simulink library "csc_gib_gdn_inertial_burn_lib"  (R2015b)
settings: Solver=ode45  StartTime=0.0  StopTime=10.0  RelTol=1e-3
values from neighbouring files (symbols this model uses):
  csc_gdn_dt = fsw_dt    [csc_gdn_guidance_init.m]
  gdn_landing_targeting_max_alt = 1000.0    (= 1000)    [csc_gdn_guidance_init.m]
  gdn_millisec_per_cycle = csc_gdn_dt*1000    [csc_gib_gdn_inertial_burn_prep.m]
undefined symbols (not defined in the file or in its folder): accel, DiscIntNeverNeededParam, pos, q, vel
libraries: util_common_lib x17, simulink x12, util_frame_rotation_lib x4, simulink_extras x3, util_info_lib x2, csu_arg_aimpoint_roll_guidance_lib x2, util_fsw_frame_rotation_lib x2, util_quat_lib x1
settings Model: Creator=Nilesh  LastModifiedBy=Mark Agbayani
settings DataIOCC: SaveFormat=Array
settings DebuggingCC: UnderspecifiedInitializationDetection=Classic  MergeDetectMultiDrivingBlocksExec=none  SolverPrmCheckMsg=warning  StateNameClashWarn=warning
settings HardwareCC: ProdBitPerPointer=32  ProdLargestAtomicFloat=None  ProdIntDivRoundTo=Undefined  ProdEndianess=Unspecified  ProdWordSize=32  ProdHWDeviceType=32-bit Generic
settings GRTTargetCC: GeneratePreprocessorConditionals=Disable all
settings ConfigComp: CovModelRefEnable=Off  CovSFcnEnable=off

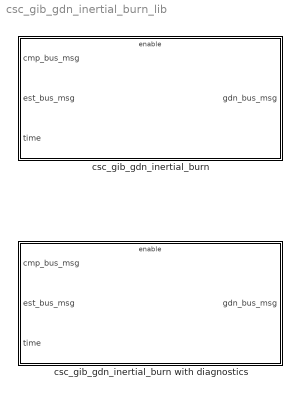
== system csc_gib_gdn_inertial_burn_lib ==
  csc_gib_gdn_inertial_burn : Subsystem
  csc_gib_gdn_inertial_burn with diagnostics : Subsystem

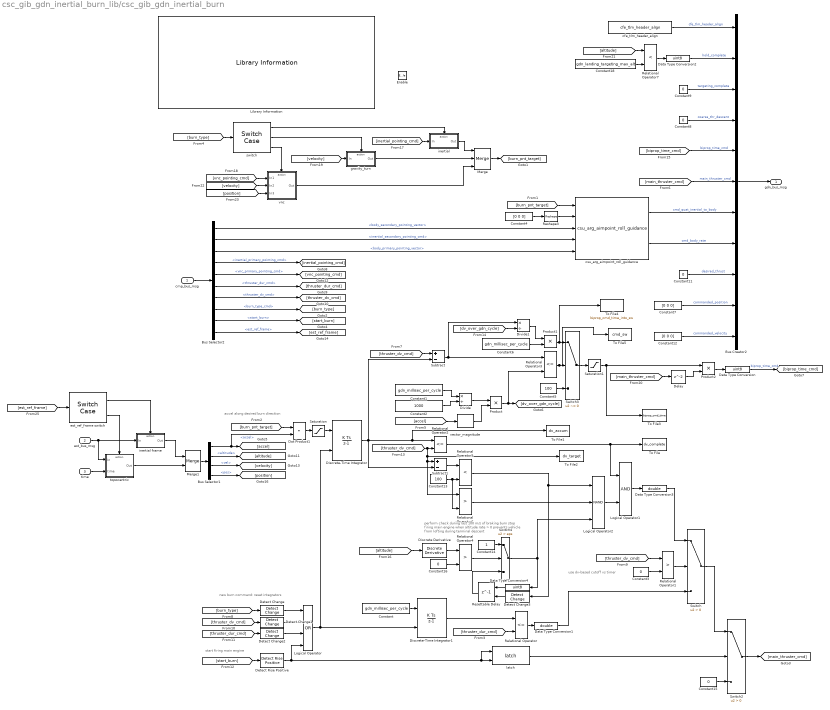
== system csc_gib_gdn_inertial_burn_lib/csc_gib_gdn_inertial_burn ==
  note: perform check during last 100 m/s of braking burn
      | stop firing main engine when altitude rate > 0
      | prevents vehicle from lofting during terminal descent
  note: use dv-based cutoff vs timer
  note: accel along desired burn direction
  note: new burn command: reset integrators
  note: start firing main engine
  cmp_bus_msg : Inport
  est_bus_msg : Inport  Port=2
  time : Inport  Port=3
  Enable : EnablePort  StatesWhenEnabling=reset
  Bus Selector1 : BusSelector  OutputSignals=accel,altitude,vel,pos
  Bus Selector2 : BusSelector  OutputSignals=body_secondary_pointing_vector,inertial_secondary_pointing_cmd,body_primary_pointing_vector,inertial_primary_pointing_cmd,vnc_primary_pointing_cmd,thruster_dur_cmd,thruster_dv_cmd,burn_type_cmd,start_burn,est_ref_frame
  Bus Creator2 : BusCreator  Inputs=11  OutDataTypeStr=Bus: gdn_bus_msg  NonVirtualBus=on
  Constant : Constant  Value=gdn_millisec_per_cycle
  Constant1 : Constant  Value=gdn_millisec_per_cycle
  Constant11 : Constant  Value=0
  Constant12 : Constant  Value=[0 0 0]
  Constant13 : Constant  Value=100
  Constant14 : Constant  OutDataTypeStr=uint8
  Constant15 : Constant  Value=0  OutDataTypeStr=double
  Constant16 : Constant  Value=0
  Constant18 : Constant  Value=gdn_landing_targeting_max_alt
  Constant2 : Constant  Value=1000
  Constant3 : Constant  Value=0
  Constant4 : Constant  Value=[0 0 0]
  Constant5 : Constant  Value=100
  Constant6 : Constant  Value=gdn_millisec_per_cycle
  Constant7 : Constant  Value=[0 0 0]
  Constant8 : Constant  Value=0  OutDataTypeStr=uint8
  Constant9 : Constant  Value=0  OutDataTypeStr=uint8
  Data Type Conversion : DataTypeConversion  OutDataTypeStr=uint8
  Data Type Conversion1 : DataTypeConversion  OutDataTypeStr=double
  Data Type Conversion2 : DataTypeConversion  OutDataTypeStr=uint8
  Data Type Conversion3 : DataTypeConversion  OutDataTypeStr=double
  Data Type Conversion4 : DataTypeConversion  OutDataTypeStr=uint8
  Delay : Delay
  Detect Change : simulink/Logic and Bit Operations/Detect Change  vinit=0  InputProcessing=Inherited  OutDataTypeStr=boolean
  Detect Change1 : simulink/Logic and Bit Operations/Detect Change  vinit=0  InputProcessing=Inherited  OutDataTypeStr=boolean
  Detect Change2 : simulink/Logic and Bit Operations/Detect Change  vinit=0  InputProcessing=Inherited  OutDataTypeStr=boolean
  Detect Change3 : simulink/Logic and Bit Operations/Detect Change  vinit=0  InputProcessing=Inherited  OutDataTypeStr=uint8
  Detect Rise Positive : simulink/Logic and Bit Operations/Detect Rise Positive  vinit=0  InputProcessing=Inherited  OutDataTypeStr=boolean
  Discrete Derivative : simulink/Discrete/Discrete Derivative  gainval=1.0  ICPrevScaledInput=0.0  InputProcessing=Inherited  OutMin=[]  OutMax=[]  OutDataType=fixdt(1, 16)  OutScaling=2^-10  DoSatur=off
  Discrete-Time Integrator : DiscreteIntegrator  ExternalReset=rising  SampleTime=csc_gdn_dt  ICPrevOutput=DiscIntNeverNeededParam  ICPrevScaledInput=DiscIntNeverNeededParam
  Discrete-Time Integrator1 : DiscreteIntegrator  ExternalReset=rising  SampleTime=csc_gdn_dt  ICPrevOutput=DiscIntNeverNeededParam  ICPrevScaledInput=DiscIntNeverNeededParam
  Divide : Product  Inputs=*/
  Divide1 : Product  Inputs=*/
  Dot Product1 : DotProduct  InputSameDT=on  OutDataTypeStr=Inherit: Inherit via internal rule
  Library Information : util_info_lib/Library Information  owner='jkaidy'
  Logical Operator : Logic  Operator=OR  Inputs=4  AllPortsSameDT=off  OutDataTypeStr=boolean
  Logical Operator1 : Logic  AllPortsSameDT=off  OutDataTypeStr=boolean
  Logical Operator2 : Logic  Operator=NAND  Inputs=3  AllPortsSameDT=off  OutDataTypeStr=boolean
  Merge : Merge  Inputs=3  InitialOutput=[0 0 1]
  Merge1 : Merge  InitialOutput=0
  Product : Product
  Product1 : Product
  Product2 : Product
  Relational Operator : RelationalOperator  Operator=<=  OutDataTypeStr=boolean
  Relational Operator1 : RelationalOperator  Operator=>  OutDataTypeStr=boolean
  Relational Operator2 : RelationalOperator  Operator=<=  OutDataTypeStr=boolean
  Relational Operator3 : RelationalOperator  Operator=<=  OutDataTypeStr=boolean
  Relational Operator4 : RelationalOperator  Operator=>  OutDataTypeStr=boolean
  Relational Operator5 : RelationalOperator  Operator=<  OutDataTypeStr=boolean
  Relational Operator6 : RelationalOperator  Operator=>  OutDataTypeStr=boolean
  Relational Operator7 : RelationalOperator  Operator=<  OutDataTypeStr=boolean
  Resettable Delay : Delay  DelayLength=1  InitialCondition=0  ExternalReset=Rising
      settings: InputPortMap=u0,r5
  Reshape3 : Reshape  OutputDimensionality=Column vector (2-D)
  Saturation : Saturate  UpperLimit=1e6  LowerLimit=0
  Saturation1 : Saturate  UpperLimit=100  LowerLimit=0
  Subtract : Sum  Inputs=+-
  Subtract1 : Sum  Inputs=+-
  Switch : Switch  Criteria=u2 > Threshold
  Switch2 : Switch  Criteria=u2 > Threshold
  Switch3 : Switch  Criteria=u2 ~= 0
  Switch4 : Switch  Criteria=u2 > Threshold  Threshold=eps
  To File : ToFile  Filename=dv_complete  MatrixName=dv_complete  SaveFormat=Timeseries
  To File1 : ToFile  Filename=dv_accum  MatrixName=dv_accum  SaveFormat=Timeseries
  To File2 : ToFile  Filename=dv_target  MatrixName=dv_target  SaveFormat=Timeseries
  To File3 : ToFile  Filename=biprop_cmd_time  MatrixName=biprop_cmd_time  SaveFormat=Timeseries
  To File4 : ToFile  Filename=biprop_cmd_time_into_sw  MatrixName=biprop_cmd_time_into_sw  SaveFormat=Timeseries
  To File5 : ToFile  Filename=cmd_sw  MatrixName=cmd_sw  SaveFormat=Timeseries
  cfe_tlm_header_align : util_common_lib/cfe_tlm_header_align
  csu_arg_aimpoint_roll_guidance : csu_arg_aimpoint_roll_guidance_lib/csu_arg_aimpoint_roll_guidance
  est_ref_frame switch : SwitchCase  CaseConditions={uint8(enum_reference_frame.inertial),uint8(enum_reference_frame.topocentric)}  ShowDefaultCase=off
  gravity_turn : Subsystem  TreatAsAtomicUnit=on
  inertial : Subsystem  TreatAsAtomicUnit=on
  inertial frame : Subsystem  TreatAsAtomicUnit=on
  latch : util_common_lib/latch  Initial_Latch=0
  switch : SwitchCase  CaseConditions={uint8(enum_burn_type.inertial),uint8(enum_burn_type.gravity_turn),uint8(enum_burn_type.vnc)}  ShowDefaultCase=off
  topocentric : Subsystem  TreatAsAtomicUnit=on
  vector_magnitude : util_common_lib/vector_magnitude  SystemSampleTime=-1
  vnc : Subsystem  TreatAsAtomicUnit=on
  gdn_bus_msg : Outport  OutDataTypeStr=Bus: gdn_bus_msg
  wires:
  Merge/1 -> [burn_pnt_target]
  Bus Selector2/4 -> [inertial_pointing_cmd]  "<inertial_primary_pointing_cmd>"
  Bus Selector2/5 -> [vnc_pointing_cmd]  "<vnc_primary_pointing_cmd>"
  [vnc_pointing_cmd] -> vnc/1(In1)
  [inertial_pointing_cmd] -> inertial/1(In)
  [burn_type] -> switch/1
  switch/3 -> vnc/Action
  inertial/1(Out) -> Merge/1
  switch/2 -> gravity_turn/Action
  gravity_turn/1(Out) -> Merge/2
  [velocity] -> gravity_turn/1(In)
  switch/1 -> inertial/Action
  Relational Operator7/1 -> Data Type Conversion2/1
  [altitude] -> Relational Operator7/1
  Constant18/1 -> Relational Operator7/2
  Bus Selector1/3 -> [velocity]  "<vel>"
  Data Type Conversion4/1 -> Resettable Delay/1
  Switch4/1 -> Data Type Conversion4/1, Logical Operator2/3
  latch/1 -> Switch2/2
  Resettable Delay/1 -> Switch4/3
  Detect Change3/1 -> Resettable Delay/2
  Constant14/1 -> Switch4/1
  Data Type Conversion3/1 -> Switch/1
  Relational Operator4/1 -> Switch4/2
  Bus Selector1/2 -> [altitude]  "<altitude>"
  Relational Operator6/1 -> Logical Operator2/2
  Discrete Derivative/1 -> Relational Operator4/1
  [altitude] -> Discrete Derivative/1
  Constant16/1 -> Relational Operator4/2
  Relational Operator5/1 -> Detect Change3/1, Logical Operator2/1
  Subtract1/1 -> Relational Operator5/1
  Constant13/1 -> Relational Operator5/2, Relational Operator6/2
  Discrete-Time Integrator/1 -> Subtract/2, To File1/1, Relational Operator2/1, Subtract1/2
  Logical Operator1/1 -> Data Type Conversion3/1
  Logical Operator2/1 -> Logical Operator1/2
  Switch2/1 -> [main_thruster_cmd]
  Constant15/1 -> Switch2/3
  Switch/1 -> Switch2/1
  Logical Operator/1 -> Discrete-Time Integrator1/2, Discrete-Time Integrator/2
  Detect Change2/1 -> Logical Operator/3
  Detect Change1/1 -> Logical Operator/2
  Detect Change/1 -> Logical Operator/1
  [thruster_dur_cmd] -> Detect Change2/1
  [thruster_dv_cmd] -> Detect Change1/1
  [burn_type] -> Detect Change/1
  [thruster_dv_cmd] -> Relational Operator1/1
  Relational Operator/1 -> Data Type Conversion1/1
  Constant3/1 -> Relational Operator1/2
  Data Type Conversion1/1 -> Switch/3
  Merge1/1 -> Bus Selector1/1
  [thruster_dv_cmd] -> Subtract1/1, Relational Operator6/1, To File2/1, Relational Operator2/2
  Relational Operator2/1 -> To File/1, Logical Operator1/1
  [thruster_dur_cmd] -> Relational Operator/2
  Dot Product1/1 -> Saturation/1
  Bus Selector1/1 -> [accel], Dot Product1/2  "<accel>"
  Discrete-Time Integrator1/1 -> Relational Operator/1
  Constant/1 -> Discrete-Time Integrator1/1
  [burn_pnt_target] -> Dot Product1/1
  Relational Operator1/1 -> Switch/2
  [start_burn] -> Detect Rise Positive/1
  Detect Rise Positive/1 -> Logical Operator/4, latch/2, latch/1
  Saturation/1 -> Discrete-Time Integrator/1
  [thruster_dv_cmd] -> Subtract/1
  Constant1/1 -> Divide/1
  Constant2/1 -> Divide/2
  Divide/1 -> Product/1
  [accel] -> vector_magnitude/1
  Product/1 -> Relational Operator3/2, [dv_over_gdn_cycle]
  Subtract/1 -> Divide1/1, Relational Operator3/1
  Relational Operator3/1 -> To File5/1, Switch3/2
  Constant5/1 -> Switch3/3
  [dv_over_gdn_cycle] -> Divide1/2
  Constant6/1 -> Product1/2
  Divide1/1 -> Product1/1
  Product1/1 -> To File4/1, Switch3/1
  Switch3/1 -> Saturation1/1
  vector_magnitude/1 -> Product/2
  Saturation1/1 -> Product2/1, To File3/1
  Data Type Conversion/1 -> [biprop_time_cmd]  "biprop_time_cmd"
  Constant7/1 -> Bus Creator2/10  "commanded_position"
  Constant12/1 -> Bus Creator2/11  "commanded_velocity"
  cfe_tlm_header_align/1 -> Bus Creator2/1  "cfe_tlm_header_align"
  Constant9/1 -> Bus Creator2/3  "targeting_complete"
  Data Type Conversion2/1 -> Bus Creator2/2  "hold_complete"
  csu_arg_aimpoint_roll_guidance/2 -> Bus Creator2/8  "cmd_body_rate"
  csu_arg_aimpoint_roll_guidance/1 -> Bus Creator2/7  "cmd_quat_inertial_to_body"
  Bus Creator2/1 -> gdn_bus_msg/1
  [main_thruster_cmd] -> Bus Creator2/6  "main_thruster_cmd"
  Constant8/1 -> Bus Creator2/4  "coarse_thr_descent"
  Constant11/1 -> Bus Creator2/9  "desired_thrust"
  Bus Selector2/9 -> [start_burn]  "<start_burn>"
  Bus Selector2/8 -> [burn_type]  "<burn_type_cmd>"
  Constant4/1 -> Reshape3/1
  Reshape3/1 -> csu_arg_aimpoint_roll_guidance/2
  Bus Selector2/3 -> csu_arg_aimpoint_roll_guidance/5  "<body_primary_pointing_vector>"
  Bus Selector2/2 -> csu_arg_aimpoint_roll_guidance/4  "<inertial_secondary_pointing_cmd>"
  Bus Selector2/1 -> csu_arg_aimpoint_roll_guidance/3  "<body_secondary_pointing_vector>"
  Bus Selector2/6 -> [thruster_dur_cmd]  "<thruster_dur_cmd>"
  Bus Selector2/7 -> [thruster_dv_cmd]  "<thruster_dv_cmd>"
  cmp_bus_msg/1 -> Bus Selector2/1
  [burn_pnt_target] -> csu_arg_aimpoint_roll_guidance/1
  [biprop_time_cmd] -> Bus Creator2/5  "biprop_time_cmd"
  vnc/1(Out) -> Merge/3
  time/1 -> topocentric/2(time)
  est_ref_frame switch/2 -> topocentric/Action
  topocentric/1(Out) -> Merge1/2
  inertial frame/1(Out) -> Merge1/1
  est_bus_msg/1 -> topocentric/1(In), inertial frame/1(In)
  est_ref_frame switch/1 -> inertial frame/Action
  [est_ref_frame] -> est_ref_frame switch/1
  Bus Selector2/10 -> [est_ref_frame]  "<est_ref_frame>"
  [position] -> vnc/3(In3)
  [velocity] -> vnc/2(In2)
  Bus Selector1/4 -> [position]  "<pos>"
  [main_thruster_cmd] -> Delay/1
  Delay/1 -> Product2/2
  Product2/1 -> Data Type Conversion/1

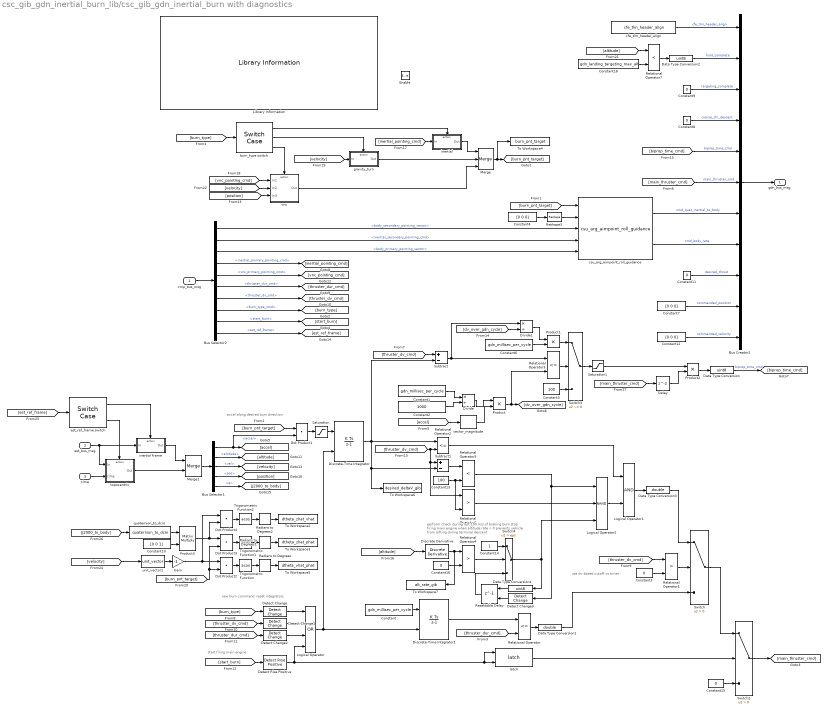
== system csc_gib_gdn_inertial_burn_lib/csc_gib_gdn_inertial_burn with diagnostics ==
  note: start firing main engine
  note: new burn command: reset integrators
  note: accel along desired burn direction
  note: use dv-based cutoff vs timer
  note: perform check during last 100 m/s of braking burn
      | stop firing main engine when altitude rate > 0
      | prevents vehicle from lofting during terminal descent
  cmp_bus_msg : Inport
  est_bus_msg : Inport  Port=2
  time : Inport  Port=3
  Enable : EnablePort  StatesWhenEnabling=reset
  Bus Selector1 : BusSelector  OutputSignals=accel,altitude,vel,pos,q
  Bus Selector2 : BusSelector  OutputSignals=body_secondary_pointing_vector,inertial_secondary_pointing_cmd,body_primary_pointing_vector,inertial_primary_pointing_cmd,vnc_primary_pointing_cmd,thruster_dur_cmd,thruster_dv_cmd,burn_type_cmd,start_burn,est_ref_frame
  Bus Creator2 : BusCreator  Inputs=11  OutDataTypeStr=Bus: gdn_bus_msg  NonVirtualBus=on
  Constant : Constant  Value=gdn_millisec_per_cycle
  Constant1 : Constant  Value=gdn_millisec_per_cycle
  Constant10 : Constant  Value=[0 0 1]
  Constant11 : Constant  Value=0
  Constant12 : Constant  Value=[0 0 0]
  Constant13 : Constant  Value=100
  Constant14 : Constant  OutDataTypeStr=uint8
  Constant15 : Constant  Value=0  OutDataTypeStr=double
  Constant16 : Constant  Value=0
  Constant18 : Constant  Value=gdn_landing_targeting_max_alt
  Constant2 : Constant  Value=1000
  Constant3 : Constant  Value=0
  Constant4 : Constant  Value=[0 0 0]
  Constant5 : Constant  Value=100
  Constant6 : Constant  Value=gdn_millisec_per_cycle
  Constant7 : Constant  Value=[0 0 0]
  Constant8 : Constant  Value=0  OutDataTypeStr=uint8
  Constant9 : Constant  Value=0  OutDataTypeStr=uint8
  Data Type Conversion : DataTypeConversion  OutDataTypeStr=uint8
  Data Type Conversion1 : DataTypeConversion  OutDataTypeStr=double
  Data Type Conversion2 : DataTypeConversion  OutDataTypeStr=uint8
  Data Type Conversion3 : DataTypeConversion  OutDataTypeStr=double
  Data Type Conversion4 : DataTypeConversion  OutDataTypeStr=uint8
  Delay : Delay
  Detect Change : simulink/Logic and Bit Operations/Detect Change  vinit=0  InputProcessing=Inherited  OutDataTypeStr=boolean
  Detect Change1 : simulink/Logic and Bit Operations/Detect Change  vinit=0  InputProcessing=Inherited  OutDataTypeStr=boolean
  Detect Change2 : simulink/Logic and Bit Operations/Detect Change  vinit=0  InputProcessing=Inherited  OutDataTypeStr=boolean
  Detect Change3 : simulink/Logic and Bit Operations/Detect Change  vinit=0  InputProcessing=Inherited  OutDataTypeStr=uint8
  Detect Rise Positive : simulink/Logic and Bit Operations/Detect Rise Positive  vinit=0  InputProcessing=Inherited  OutDataTypeStr=boolean
  Discrete Derivative : simulink/Discrete/Discrete Derivative  gainval=1.0  ICPrevScaledInput=0.0  InputProcessing=Inherited  OutMin=[]  OutMax=[]  OutDataType=fixdt(1, 16)  OutScaling=2^-10  DoSatur=off
  Discrete-Time Integrator : DiscreteIntegrator  ExternalReset=rising  SampleTime=csc_gdn_dt  ICPrevOutput=DiscIntNeverNeededParam  ICPrevScaledInput=DiscIntNeverNeededParam
  Discrete-Time Integrator1 : DiscreteIntegrator  ExternalReset=rising  SampleTime=csc_gdn_dt  ICPrevOutput=DiscIntNeverNeededParam  ICPrevScaledInput=DiscIntNeverNeededParam
  Divide : Product  Inputs=*/
  Divide1 : Product  Inputs=*/
  Dot Product{1..4} (4 alike) : DotProduct  InputSameDT=on  OutDataTypeStr=Inherit: Inherit via internal rule
  Gain : Gain  Gain=-1
  Library Information : util_info_lib/Library Information  owner='jkaidy'
  Logical Operator : Logic  Operator=OR  Inputs=4  AllPortsSameDT=off  OutDataTypeStr=boolean
  Logical Operator1 : Logic  AllPortsSameDT=off  OutDataTypeStr=boolean
  Logical Operator2 : Logic  Operator=NAND  Inputs=3  AllPortsSameDT=off  OutDataTypeStr=boolean
  Merge : Merge  Inputs=3  InitialOutput=[0 0 1]
  Merge1 : Merge  InitialOutput=0
  Product : Product
  Product1 : Product
  Product2 : Product
  Product3 : Product  Multiplication=Matrix(*)  RndMeth=Zero
  Radians to Degrees : simulink_extras/Transformations/Radians to Degrees
  Radians to Degrees1 : simulink_extras/Transformations/Radians to Degrees
  Radians to Degrees2 : simulink_extras/Transformations/Radians to Degrees
  Relational Operator : RelationalOperator  Operator=<=  OutDataTypeStr=boolean
  Relational Operator1 : RelationalOperator  Operator=>  OutDataTypeStr=boolean
  Relational Operator2 : RelationalOperator  Operator=<=  OutDataTypeStr=boolean
  Relational Operator3 : RelationalOperator  Operator=<=  OutDataTypeStr=boolean
  Relational Operator4 : RelationalOperator  Operator=>  OutDataTypeStr=boolean
  Relational Operator5 : RelationalOperator  Operator=<  OutDataTypeStr=boolean
  Relational Operator6 : RelationalOperator  Operator=>  OutDataTypeStr=boolean
  Relational Operator7 : RelationalOperator  Operator=<  OutDataTypeStr=boolean
  Resettable Delay : Delay  DelayLength=1  InitialCondition=0  ExternalReset=Rising
      settings: InputPortMap=u0,r5
  Reshape3 : Reshape  OutputDimensionality=Column vector (2-D)
  Saturation : Saturate  UpperLimit=1e6  LowerLimit=0
  Saturation1 : Saturate  UpperLimit=100  LowerLimit=0
  Subtract : Sum  Inputs=+-
  Subtract1 : Sum  Inputs=+-
  Switch : Switch  Criteria=u2 > Threshold
  Switch2 : Switch  Criteria=u2 > Threshold
  Switch3 : Switch  Criteria=u2 ~= 0
  Switch4 : Switch  Criteria=u2 > Threshold  Threshold=eps
  To Workspace2 : ToWorkspace  VariableName=dtheta_zhat_vhat  SaveFormat=Structure With Time  SampleTime=-1
  To Workspace3 : ToWorkspace  VariableName=dtheta_zhat_phat  SaveFormat=Structure With Time  SampleTime=-1
  To Workspace4 : ToWorkspace  VariableName=burn_pnt_target  SaveFormat=Structure With Time  SampleTime=-1
  To Workspace5 : ToWorkspace  VariableName=dtheta_vhat_phat  SaveFormat=Structure With Time  SampleTime=-1
  To Workspace6 : ToWorkspace  VariableName=desired_deltaV_gib  SaveFormat=Structure With Time  SampleTime=-1
  To Workspace7 : ToWorkspace  VariableName=alt_rate_gib  SaveFormat=Structure With Time  SampleTime=-1
  Trigonometric Function : Trigonometry  Operator=acos
  Trigonometric Function1 : Trigonometry  Operator=acos
  Trigonometric Function2 : Trigonometry  Operator=acos
  burn_type switch : SwitchCase  CaseConditions={uint8(enum_burn_type.inertial),uint8(enum_burn_type.gravity_turn),uint8(enum_burn_type.vnc)}  ShowDefaultCase=off
  cfe_tlm_header_align : util_common_lib/cfe_tlm_header_align
  csu_arg_aimpoint_roll_guidance : csu_arg_aimpoint_roll_guidance_lib/csu_arg_aimpoint_roll_guidance
  est_ref_frame switch : SwitchCase  CaseConditions={uint8(enum_reference_frame.inertial),uint8(enum_reference_frame.topocentric)}  ShowDefaultCase=off
  gravity_turn : Subsystem  TreatAsAtomicUnit=on
  inertial : Subsystem  TreatAsAtomicUnit=on
  inertial frame : Subsystem  TreatAsAtomicUnit=on
  latch : util_common_lib/latch  Initial_Latch=0
  quaternion_to_dcm : util_quat_lib/quaternion_to_dcm  SystemSampleTime=-1
  topocentric : Subsystem  TreatAsAtomicUnit=on
  unit_vector1 : util_common_lib/unit_vector  SystemSampleTime=-1
  vector_magnitude : util_common_lib/vector_magnitude  SystemSampleTime=-1
  vnc : Subsystem  TreatAsAtomicUnit=on
  gdn_bus_msg : Outport  OutDataTypeStr=Bus: gdn_bus_msg
  wires:
  Product2/1 -> Data Type Conversion/1
  Delay/1 -> Product2/2
  [main_thruster_cmd] -> Delay/1
  Data Type Conversion/1 -> [biprop_time_cmd]  "biprop_time_cmd"
  Saturation1/1 -> Product2/1
  Bus Selector1/5 -> [J2000_to_body]  "<q>"
  [velocity] -> vnc/2(In2)
  [position] -> vnc/3(In3)
  Bus Selector1/4 -> [position]  "<pos>"
  vnc/1(Out) -> Merge/3
  [biprop_time_cmd] -> Bus Creator2/5  "biprop_time_cmd"
  [burn_pnt_target] -> csu_arg_aimpoint_roll_guidance/1
  cmp_bus_msg/1 -> Bus Selector2/1
  Bus Selector2/7 -> [thruster_dv_cmd]  "<thruster_dv_cmd>"
  Bus Selector2/6 -> [thruster_dur_cmd]  "<thruster_dur_cmd>"
  Bus Selector2/1 -> csu_arg_aimpoint_roll_guidance/3  "<body_secondary_pointing_vector>"
  Bus Selector2/2 -> csu_arg_aimpoint_roll_guidance/4  "<inertial_secondary_pointing_cmd>"
  Bus Selector2/3 -> csu_arg_aimpoint_roll_guidance/5  "<body_primary_pointing_vector>"
  Reshape3/1 -> csu_arg_aimpoint_roll_guidance/2
  Constant4/1 -> Reshape3/1
  Bus Selector2/8 -> [burn_type]  "<burn_type_cmd>"
  Bus Selector2/9 -> [start_burn]  "<start_burn>"
  Constant11/1 -> Bus Creator2/9  "desired_thrust"
  Constant8/1 -> Bus Creator2/4  "coarse_thr_descent"
  [main_thruster_cmd] -> Bus Creator2/6  "main_thruster_cmd"
  Bus Creator2/1 -> gdn_bus_msg/1
  csu_arg_aimpoint_roll_guidance/1 -> Bus Creator2/7  "cmd_quat_inertial_to_body"
  csu_arg_aimpoint_roll_guidance/2 -> Bus Creator2/8  "cmd_body_rate"
  Data Type Conversion2/1 -> Bus Creator2/2  "hold_complete"
  Constant9/1 -> Bus Creator2/3  "targeting_complete"
  cfe_tlm_header_align/1 -> Bus Creator2/1  "cfe_tlm_header_align"
  Constant12/1 -> Bus Creator2/11  "commanded_velocity"
  Constant7/1 -> Bus Creator2/10  "commanded_position"
  vector_magnitude/1 -> Product/2
  Switch3/1 -> Saturation1/1
  Product1/1 -> Switch3/1
  Divide1/1 -> Product1/1
  Constant6/1 -> Product1/2
  [dv_over_gdn_cycle] -> Divide1/2
  Constant5/1 -> Switch3/3
  Relational Operator3/1 -> Switch3/2
  Subtract/1 -> Relational Operator3/1, Divide1/1
  Product/1 -> [dv_over_gdn_cycle], Relational Operator3/2
  [accel] -> vector_magnitude/1
  Divide/1 -> Product/1
  Constant2/1 -> Divide/2
  Constant1/1 -> Divide/1
  [thruster_dv_cmd] -> Subtract/1
  Saturation/1 -> Discrete-Time Integrator/1
  Detect Rise Positive/1 -> latch/1, latch/2, Logical Operator/4
  [start_burn] -> Detect Rise Positive/1
  Relational Operator1/1 -> Switch/2
  [burn_pnt_target] -> Dot Product1/1
  Constant/1 -> Discrete-Time Integrator1/1
  Discrete-Time Integrator1/1 -> Relational Operator/1
  Bus Selector1/1 -> Dot Product1/2, [accel]  "<accel>"
  Dot Product1/1 -> Saturation/1
  [thruster_dur_cmd] -> Relational Operator/2
  Relational Operator2/1 -> Logical Operator1/1
  [thruster_dv_cmd] -> Relational Operator6/1, Subtract1/1, Relational Operator2/2
  Data Type Conversion1/1 -> Switch/3
  Constant3/1 -> Relational Operator1/2
  Relational Operator/1 -> Data Type Conversion1/1
  [thruster_dv_cmd] -> Relational Operator1/1
  [burn_type] -> Detect Change/1
  [thruster_dv_cmd] -> Detect Change1/1
  [thruster_dur_cmd] -> Detect Change2/1
  Detect Change/1 -> Logical Operator/1
  Detect Change1/1 -> Logical Operator/2
  Detect Change2/1 -> Logical Operator/3
  Logical Operator/1 -> Discrete-Time Integrator/2, Discrete-Time Integrator1/2
  Switch/1 -> Switch2/1
  Constant15/1 -> Switch2/3
  Switch2/1 -> [main_thruster_cmd]
  Logical Operator2/1 -> Logical Operator1/2
  Logical Operator1/1 -> Data Type Conversion3/1
  Discrete-Time Integrator/1 -> Subtract1/2, To Workspace6/1, Subtract/2, Relational Operator2/1
  Constant13/1 -> Relational Operator6/2, Relational Operator5/2
  Subtract1/1 -> Relational Operator5/1
  Relational Operator5/1 -> Logical Operator2/1, Detect Change3/1
  Constant16/1 -> Relational Operator4/2
  [altitude] -> Discrete Derivative/1
  Discrete Derivative/1 -> To Workspace7/1, Relational Operator4/1
  Relational Operator6/1 -> Logical Operator2/2
  Bus Selector1/2 -> [altitude]  "<altitude>"
  Relational Operator4/1 -> Switch4/2
  Data Type Conversion3/1 -> Switch/1
  Constant14/1 -> Switch4/1
  Detect Change3/1 -> Resettable Delay/2
  Resettable Delay/1 -> Switch4/3
  latch/1 -> Switch2/2
  Switch4/1 -> Logical Operator2/3, Data Type Conversion4/1
  Data Type Conversion4/1 -> Resettable Delay/1
  Bus Selector1/3 -> [velocity]  "<vel>"
  Product3/1 -> Dot Product3/1, Dot Product4/2
  Trigonometric Function1/1 -> Radians to Degrees1/1
  Dot Product3/1 -> Trigonometric Function1/1
  Constant10/1 -> Product3/2
  quaternion_to_dcm/1 -> Product3/1
  [J2000_to_body] -> quaternion_to_dcm/1
  Gain/1 -> Dot Product4/1, Dot Product2/1
  Trigonometric Function/1 -> Radians to Degrees/1
  Dot Product2/1 -> Trigonometric Function/1
  unit_vector1/1 -> Gain/1
  [velocity] -> unit_vector1/1
  [burn_pnt_target] -> Dot Product2/2, Dot Product3/2
  Trigonometric Function2/1 -> Radians to Degrees2/1
  Dot Product4/1 -> Trigonometric Function2/1
  Radians to Degrees2/1 -> To Workspace2/1
  Radians to Degrees1/1 -> To Workspace3/1
  Radians to Degrees/1 -> To Workspace5/1
  Constant18/1 -> Relational Operator7/2
  [altitude] -> Relational Operator7/1
  Relational Operator7/1 -> Data Type Conversion2/1
  burn_type switch/1 -> inertial/Action
  [velocity] -> gravity_turn/1(In)
  gravity_turn/1(Out) -> Merge/2
  burn_type switch/2 -> gravity_turn/Action
  inertial/1(Out) -> Merge/1
  burn_type switch/3 -> vnc/Action
  [burn_type] -> burn_type switch/1
  [inertial_pointing_cmd] -> inertial/1(In)
  [vnc_pointing_cmd] -> vnc/1(In1)
  Bus Selector2/5 -> [vnc_pointing_cmd]  "<vnc_primary_pointing_cmd>"
  Bus Selector2/4 -> [inertial_pointing_cmd]  "<inertial_primary_pointing_cmd>"
  Merge/1 -> To Workspace4/1, [burn_pnt_target]
  [est_ref_frame] -> est_ref_frame switch/1
  est_ref_frame switch/1 -> inertial frame/Action
  est_bus_msg/1 -> topocentric/1(In), inertial frame/1(In)
  inertial frame/1(Out) -> Merge1/1
  topocentric/1(Out) -> Merge1/2
  est_ref_frame switch/2 -> topocentric/Action
  Merge1/1 -> Bus Selector1/1
  time/1 -> topocentric/2(time)
  Bus Selector2/10 -> [est_ref_frame]  "<est_ref_frame>"

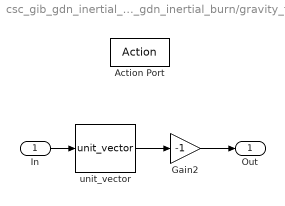
== system csc_gib_gdn_inertial_burn_lib/csc_gib_gdn_inertial_burn/gravity_turn ==
  In : Inport
  Action Port : ActionPort
  Gain2 : Gain  Gain=-1
  unit_vector : util_common_lib/unit_vector  SystemSampleTime=-1
  Out : Outport
  wires:
  Gain2/1 -> Out/1
  unit_vector/1 -> Gain2/1
  In/1 -> unit_vector/1

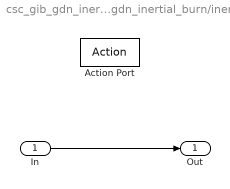
== system csc_gib_gdn_inertial_burn_lib/csc_gib_gdn_inertial_burn/inertial ==
  In : Inport
  Action Port : ActionPort
  Out : Outport
  wires:
  In/1 -> Out/1

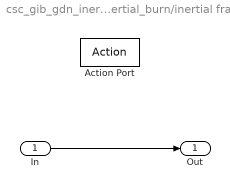
== system csc_gib_gdn_inertial_burn_lib/csc_gib_gdn_inertial_burn/inertial frame ==
  In : Inport
  Action Port : ActionPort
  Out : Outport
  wires:
  In/1 -> Out/1

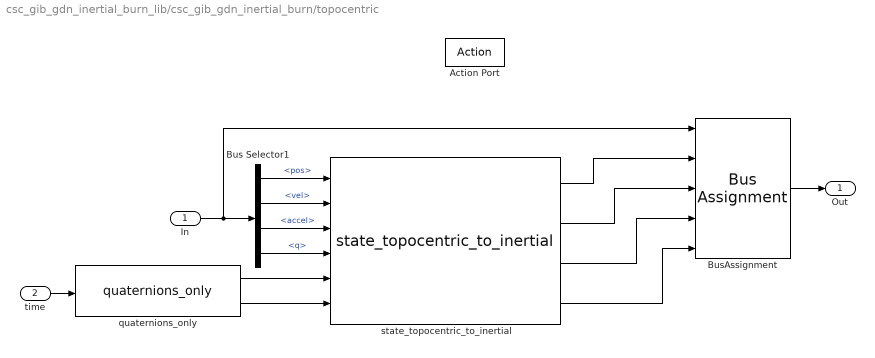
== system csc_gib_gdn_inertial_burn_lib/csc_gib_gdn_inertial_burn/topocentric ==
  In : Inport
  time : Inport  Port=2
  Action Port : ActionPort  ActionType=case
  Bus Selector1 : BusSelector  OutputSignals=pos,vel,accel,q
  BusAssignment : BusAssignment  AssignedSignals=pos,vel,accel,q
  quaternions_only : util_frame_rotation_lib/quaternions_only  SystemSampleTime=-1
  state_topocentric_to_inertial : util_fsw_frame_rotation_lib/state_topocentric_to_inertial  SystemSampleTime=-1
  Out : Outport
  wires:
  state_topocentric_to_inertial/4 -> BusAssignment/5
  Bus Selector1/4 -> state_topocentric_to_inertial/4  "<q>"
  Bus Selector1/1 -> state_topocentric_to_inertial/1  "<pos>"
  Bus Selector1/2 -> state_topocentric_to_inertial/2  "<vel>"
  Bus Selector1/3 -> state_topocentric_to_inertial/3  "<accel>"
  In/1 -> BusAssignment/1, Bus Selector1/1
  state_topocentric_to_inertial/1 -> BusAssignment/2
  state_topocentric_to_inertial/2 -> BusAssignment/3
  state_topocentric_to_inertial/3 -> BusAssignment/4
  BusAssignment/1 -> Out/1
  time/1 -> quaternions_only/1
  quaternions_only/1 -> state_topocentric_to_inertial/5
  quaternions_only/2 -> state_topocentric_to_inertial/6

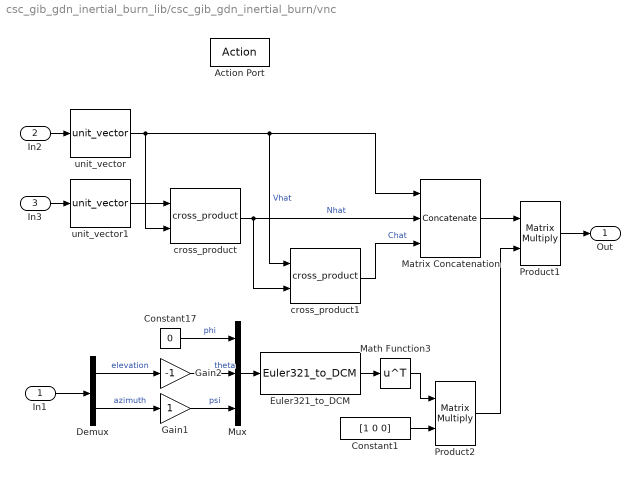
== system csc_gib_gdn_inertial_burn_lib/csc_gib_gdn_inertial_burn/vnc ==
  In1 : Inport
  In2 : Inport  Port=2
  In3 : Inport  Port=3
  Action Port : ActionPort  ActionType=case
  Constant1 : Constant  Value=[1 0 0]
  Constant17 : Constant  Value=0  OutDataTypeStr=double
  Demux : Demux  Outputs=2
  Euler321_to_DCM : util_frame_rotation_lib/Euler321_to_DCM
  Gain1 : Gain
  Gain2 : Gain  Gain=-1
  Math Function3 : Math  Operator=transpose  SaturateOnIntegerOverflow=on
  Matrix Concatenation : Concatenate  NumInputs=3  Mode=Multidimensional array  ConcatenateDimension=2
  Mux : Mux  Inputs=3
  Product1 : Product  Multiplication=Matrix(*)
  Product2 : Product  Multiplication=Matrix(*)
  cross_product : util_common_lib/cross_product  SystemSampleTime=-1
  cross_product1 : util_common_lib/cross_product  SystemSampleTime=-1
  unit_vector : util_common_lib/unit_vector  SystemSampleTime=-1
  unit_vector1 : util_common_lib/unit_vector  SystemSampleTime=-1
  Out : Outport
  wires:
  Product2/1 -> Product1/2
  Product1/1 -> Out/1
  Constant1/1 -> Product2/2
  Matrix Concatenation/1 -> Product1/1
  unit_vector1/1 -> cross_product/1
  cross_product1/1 -> Matrix Concatenation/3  "Chat"
  cross_product/1 -> Matrix Concatenation/2, cross_product1/2  "Nhat"
  unit_vector/1 -> Matrix Concatenation/1, cross_product1/1, cross_product/2  "Vhat"
  In3/1 -> unit_vector1/1
  Mux/1 -> Euler321_to_DCM/1
  Euler321_to_DCM/1 -> Math Function3/1
  Constant17/1 -> Mux/1  "phi"
  Gain1/1 -> Mux/3  "psi"
  Gain2/1 -> Mux/2  "theta"
  In2/1 -> unit_vector/1
  In1/1 -> Demux/1
  Demux/1 -> Gain2/1  "elevation"
  Demux/2 -> Gain1/1  "azimuth"
  Math Function3/1 -> Product2/1

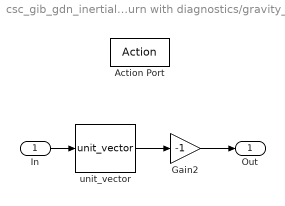
== system csc_gib_gdn_inertial_burn_lib/csc_gib_gdn_inertial_burn with diagnostics/gravity_turn ==
  In : Inport
  Action Port : ActionPort
  Gain2 : Gain  Gain=-1
  unit_vector : util_common_lib/unit_vector  SystemSampleTime=-1
  Out : Outport
  wires:
  In/1 -> unit_vector/1
  unit_vector/1 -> Gain2/1
  Gain2/1 -> Out/1

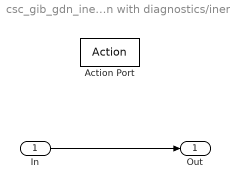
== system csc_gib_gdn_inertial_burn_lib/csc_gib_gdn_inertial_burn with diagnostics/inertial ==
  In : Inport
  Action Port : ActionPort
  Out : Outport
  wires:
  In/1 -> Out/1

== system csc_gib_gdn_inertial_burn_lib/csc_gib_gdn_inertial_burn with diagnostics/inertial frame ==
  In : Inport
  Action Port : ActionPort
  Out : Outport
  wires:
  In/1 -> Out/1

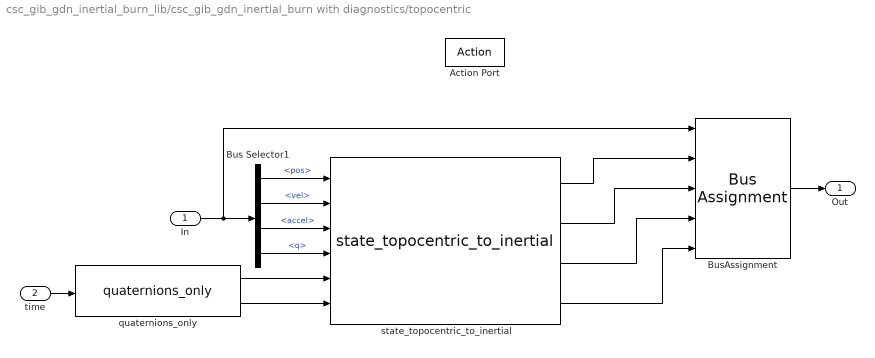
== system csc_gib_gdn_inertial_burn_lib/csc_gib_gdn_inertial_burn with diagnostics/topocentric ==
  In : Inport
  time : Inport  Port=2
  Action Port : ActionPort
  Bus Selector1 : BusSelector  OutputSignals=pos,vel,accel,q
  BusAssignment : BusAssignment  AssignedSignals=pos,vel,accel,q
  quaternions_only : util_frame_rotation_lib/quaternions_only  SystemSampleTime=-1
  state_topocentric_to_inertial : util_fsw_frame_rotation_lib/state_topocentric_to_inertial  SystemSampleTime=-1
  Out : Outport
  wires:
  state_topocentric_to_inertial/4 -> BusAssignment/5
  Bus Selector1/4 -> state_topocentric_to_inertial/4  "<q>"
  Bus Selector1/1 -> state_topocentric_to_inertial/1  "<pos>"
  Bus Selector1/2 -> state_topocentric_to_inertial/2  "<vel>"
  Bus Selector1/3 -> state_topocentric_to_inertial/3  "<accel>"
  In/1 -> BusAssignment/1, Bus Selector1/1
  state_topocentric_to_inertial/1 -> BusAssignment/2
  state_topocentric_to_inertial/2 -> BusAssignment/3
  state_topocentric_to_inertial/3 -> BusAssignment/4
  BusAssignment/1 -> Out/1
  time/1 -> quaternions_only/1
  quaternions_only/1 -> state_topocentric_to_inertial/5
  quaternions_only/2 -> state_topocentric_to_inertial/6

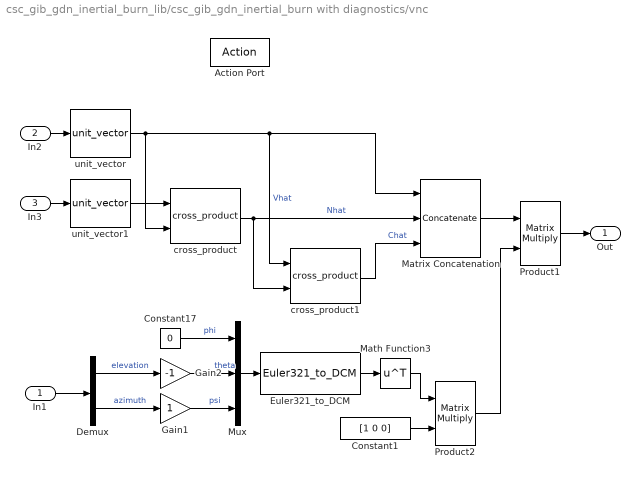
== system csc_gib_gdn_inertial_burn_lib/csc_gib_gdn_inertial_burn with diagnostics/vnc ==
  In1 : Inport
  In2 : Inport  Port=2
  In3 : Inport  Port=3
  Action Port : ActionPort
  Constant1 : Constant  Value=[1 0 0]
  Constant17 : Constant  Value=0  OutDataTypeStr=double
  Demux : Demux  Outputs=2
  Euler321_to_DCM : util_frame_rotation_lib/Euler321_to_DCM
  Gain1 : Gain
  Gain2 : Gain  Gain=-1
  Math Function3 : Math  Operator=transpose  SaturateOnIntegerOverflow=on
  Matrix Concatenation : Concatenate  NumInputs=3  Mode=Multidimensional array  ConcatenateDimension=2
  Mux : Mux  Inputs=3
  Product1 : Product  Multiplication=Matrix(*)
  Product2 : Product  Multiplication=Matrix(*)
  cross_product : util_common_lib/cross_product  SystemSampleTime=-1
  cross_product1 : util_common_lib/cross_product  SystemSampleTime=-1
  unit_vector : util_common_lib/unit_vector  SystemSampleTime=-1
  unit_vector1 : util_common_lib/unit_vector  SystemSampleTime=-1
  Out : Outport
  wires:
  Math Function3/1 -> Product2/1
  Demux/2 -> Gain1/1  "azimuth"
  Demux/1 -> Gain2/1  "elevation"
  In1/1 -> Demux/1
  In2/1 -> unit_vector/1
  Gain2/1 -> Mux/2  "theta"
  Gain1/1 -> Mux/3  "psi"
  Constant17/1 -> Mux/1  "phi"
  Euler321_to_DCM/1 -> Math Function3/1
  Mux/1 -> Euler321_to_DCM/1
  In3/1 -> unit_vector1/1
  unit_vector/1 -> cross_product/2, cross_product1/1, Matrix Concatenation/1  "Vhat"
  cross_product/1 -> cross_product1/2, Matrix Concatenation/2  "Nhat"
  cross_product1/1 -> Matrix Concatenation/3  "Chat"
  unit_vector1/1 -> cross_product/1
  Matrix Concatenation/1 -> Product1/1
  Constant1/1 -> Product2/2
  Product1/1 -> Out/1
  Product2/1 -> Product1/2
